simulink model "M53"  (R2021b)
settings: Solver=VariableStepAuto  StartTime=0.0  StopTime=10.0  RelTol=1e-3
settings Model: Creator=abdul  LastModifiedBy=abdul

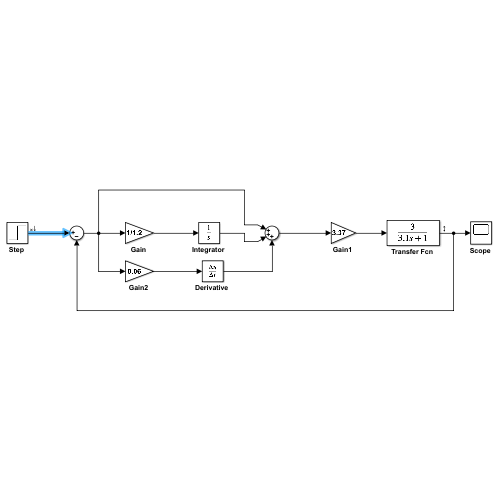
[thumbnail: Simulink's stored preview of the top-level diagram]
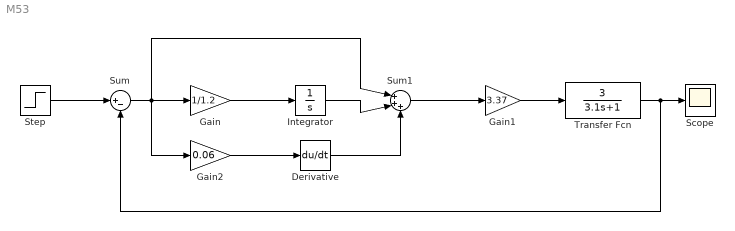
== system M53 ==
  "Derivative " : Derivative
  "Gain " : Gain  Gain=1/1.2
  "Gain1 " : Gain  Gain=3.37
  "Gain2 " : Gain  Gain=0.06
  "Integrator " : Integrator
  "Scope " : Scope
  "Step " : Step  Time=0  After=30  SampleTime=0
  Sum : Sum  Inputs=|+-
  Sum1 : Sum  Inputs=|+++
  "Transfer Fcn " : TransferFcn  Numerator=[3]  Denominator=[3.1 1]
  wires:
  "Step "/1 -> Sum/1
  Sum/1 -> Sum1/1, "Gain2 "/1, "Gain "/1
  "Gain "/1 -> "Integrator "/1
  "Gain2 "/1 -> "Derivative "/1
  "Integrator "/1 -> Sum1/2
  "Derivative "/1 -> Sum1/3
  Sum1/1 -> "Gain1 "/1
  "Gain1 "/1 -> "Transfer Fcn "/1
  "Transfer Fcn "/1 -> Sum/2, "Scope "/1
